simulink model "spectrum_analysis_model"  (R2024b)
settings: Solver=VariableStepAuto  StartTime=0.0  StopTime=10.0  RelTol=1e-3
settings Model: Creator=castl  LastModifiedBy=castl

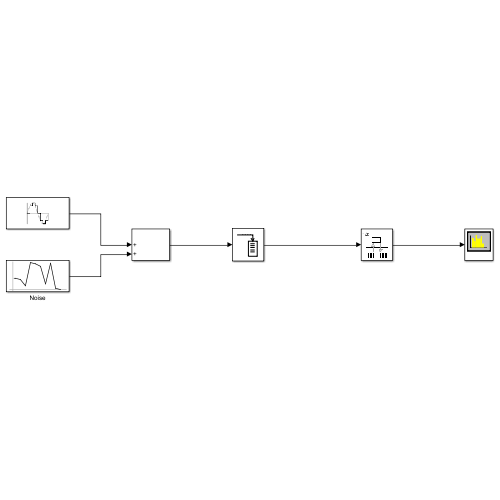
[thumbnail: Simulink's stored preview of the top-level diagram]
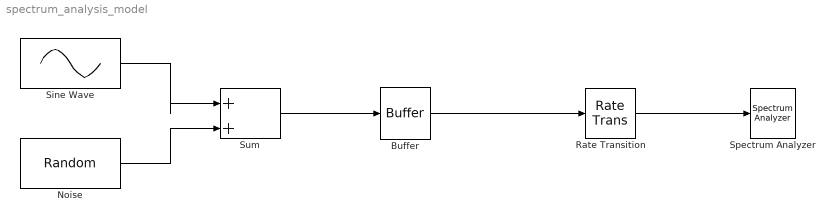
== system spectrum_analysis_model ==
  Buffer : Buffer  N=1024  OutputFrames=off
  Noise : RandomNumber  Variance=0.2  SampleTime=0.001
  Rate Transition : RateTransition
  Sine Wave : Sin  Frequency=50  SampleTime=0.001
  Spectrum Analyzer : SpectrumAnalyzer  WindowPosition=[880.000000,470.000000,800.000000,500.000000,]  ScopeFrameLocation=window  Method=Welch  FrequencyResolutionMethod=Window length  WindowInvariantSamplesPerUpdate=on  YLimits=[-2118.287664939324,1755.3679089298919]  SelectedToolstripTab=spectrumAnalyzerToolstrip.estimationTab
  Sum : Sum  Inputs=|++
  wires:
  Sum/1 -> Buffer/1
  Noise/1 -> Sum/2
  Sine Wave/1 -> Sum/1
  Rate Transition/1 -> Spectrum Analyzer/1
  Buffer/1 -> Rate Transition/1
